simulink model "ssTest1"  (R2023b)
settings: Solver=VariableStepAuto  StartTime=0.0  StopTime=10.0  RelTol=1e-3
values from neighbouring files (symbols this model uses):
  Ad1 = A    [cDQN.m]    (also in ssTest.m = INVR*(I+A*dt/2))
  B = A*X    [Copy_of_cDQN.m]    (also in cCOM.m; cDQN.m)
  Bd1 = B    [cDQN.m]    (also in ssTest.m = INVR*B*dt/2)
  C = obj.fCalcMat(X(1)+1i*X(2) , B(1)+1i*B(2))    [Copy_of_cDQN.m]    (also in cCOM.m; cDQN.m)
  Cd1 = C    [cDQN.m]    (also in ssTest.m = C*Ad1)
  Dd11 = C*INVR*B*dt/2+D    [ssTest.m]
  Dd12 = C*INVR*B*dt/2    [ssTest.m]
undefined symbols (not defined in the file or in its folder): A, Ad2, Ad3, Bd2, Bd3, Cd21, Cd22, Cd3, D, Dd2, Dd3, Ts
libraries: DQN_Lib x1, spspowerguiLib x1
settings Model: Creator=rober  LastModifiedBy=rober

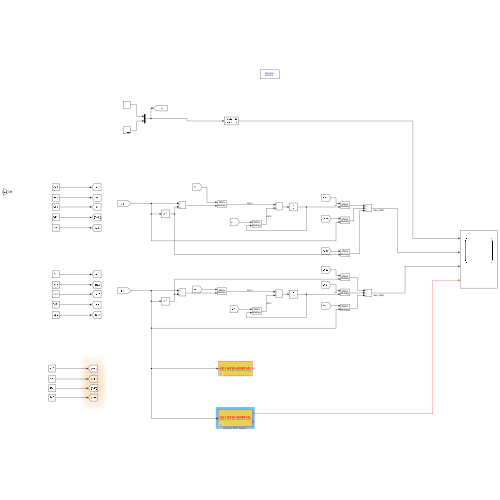
[thumbnail: Simulink's stored preview of the top-level diagram]
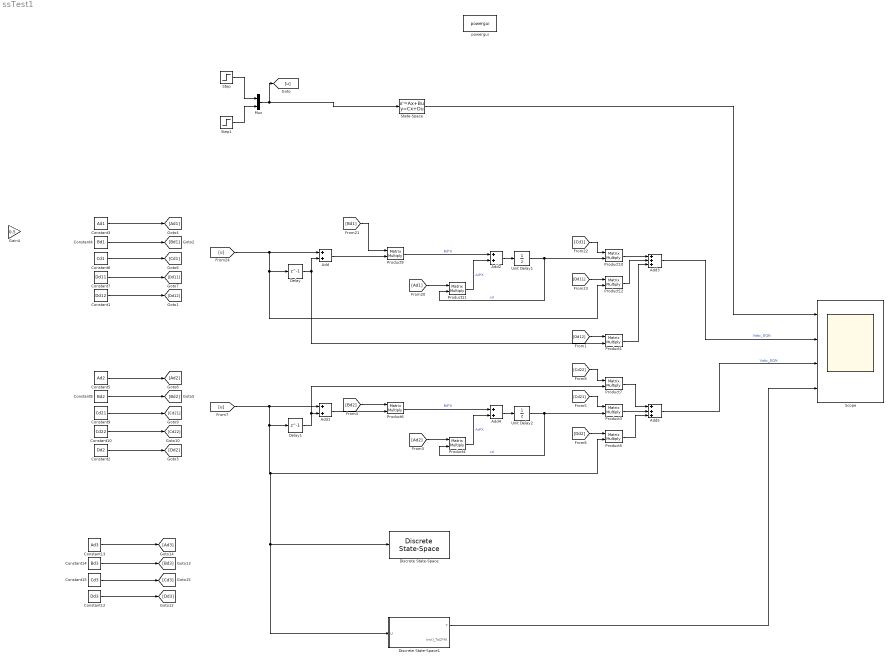
== system ssTest1 ==
  Add{,1..2,4} (4 alike) : Sum
  Add3 : Sum  Inputs=+++
  Add5 : Sum  Inputs=+++
  Constant1 : Constant  Value=Dd12
  Constant10 : Constant  Value=Cd22
  Constant12 : Constant  Value=Dd3
  Constant13 : Constant  Value=Ad3
  Constant14 : Constant  Value=Bd3
  Constant15 : Constant  Value=Cd3
  Constant2 : Constant  Value=Dd2
  Constant3 : Constant  Value=Ad1
  Constant4 : Constant  Value=Bd1
  Constant5 : Constant  Value=Ad2
  Constant6 : Constant  Value=Cd1
  Constant7 : Constant  Value=Dd11
  Constant8 : Constant  Value=Bd2
  Constant9 : Constant  Value=Cd21
  Delay : Delay  DelayLength=1  SampleTime=Ts
  Delay1 : Delay  DelayLength=1  SampleTime=Ts
  Discrete State-Space : DQN_Lib/Discrete State-Space  A=A  B=B  C=C  D=D  InitVec=0  dt=Ts
      settings: LibrarySourceBlock=|
      | spsSynchronousMachineModel/Discrete robust/State Space Model/Discretize
      | BE or Tustin
  Discrete State-Space1 : Subsystem  mask{A=A, B=B, C=C, D=D, InitVec=0, dt=Ts}
      mask prompts: InitVec "Initial condition:"; dt "Time step (s):"
      mask init:
      | I = eye(size(A,1));
      | INVR = I/(I-A*dt/2);
      | Ad1 = INVR*(I+A*dt/2);
      | Bd1 = INVR*B*dt/2;
      | Cd1 = C*Ad1;
      | Dd11 = C*INVR*B*dt/2+D;
      | Dd12 = C*INVR*B*dt/2;
      settings: LibrarySourceBlock=|
      | spsSynchronousMachineModel/Discrete robust/State Space Model/Discretize
      | BE or Tustin
      mask Display: disp(['{\color{red}\bf\fontsize{12}x(t) = Ad*x(t-dt)+Bd*u(t)}',newline,'{\color{gray}\bf\fontsize{12}y(t) = Cd*x(t-dt)+Dd*u(t)}'], 'texmode','on');
  Gain4 : Gain  Gain=0.5
  Mux : Mux  Inputs=2
  Product{1,3..7,9..12} (10 alike) : Product  Multiplication=Matrix(*)  SaturateOnIntegerOverflow=on  OutDataTypeStr=Inherit: Same as first input
  Scope : Scope  NumInputPorts=4
  State-Space : StateSpace  A=A  B=B  C=C  D=D  InitialCondition=0
  Step : Step  Time=3  Before=-0.668  After=5.668  SampleTime=Ts
  Step1 : Step  Time=8  Before=3.668  After=1.854  SampleTime=Ts
  Unit Delay1 : UnitDelay  SampleTime=Ts  HasFrameUpgradeWarning=on
  Unit Delay2 : UnitDelay  SampleTime=Ts  HasFrameUpgradeWarning=on
  powergui : spspowerguiLib/powergui  Priority=1  SimulationMode=Discrete  SampleTime=Ts  frequency=60  Iterations=50  frequencyindice=60  Pbase=100e6  ErrMax=1e-4  UnitsV=kV  UnitsW=MW  buscounter=0  FunctionMessages=off  echomessages=off  EnableUseOfTLC=off  CurrentSourceSwitches=off  DisableSnubberDevices=off  DisableRonSwitches=off  DisableVfSwitches=off  DisplayEquations=off  AutomaticDiscreteSolvers=off  SolverType=Tustin/Backward Euler (TBE)  Interpol=off  ExternalGateDelay=off  methode=off  Ts=100  x0status=blocks  SPID=on  SwTol=0  HookPort=off  NonlinearTolerance=1e-4  nMaxIteration=100  ContinueOnMaxIteration=off  RestoreLinks=warning  ResistiveCurrentMeasurement=off  Frange=[0:2:500]  Ylog=off  Xlog=on  ShowGrid=off  save=off  variable=ZData  structure=0  ZoomFFT=off  StartTime=0.0  cycles=1  DisplayStyle=1  fundamental=60  FreqAxis=off  MaxFrequency=1000  frequencyindicesteady=1  RmsSteady=1  display=off
  wires:
  Mux/1 -> [u], State-Space/1
  Step/1 -> Mux/1
  Step1/1 -> Mux/2
  State-Space/1 -> Scope/1
  Product10/1 -> Add3/1
  [Cd1] -> Product10/1
  Add/1 -> Product9/2
  Constant6/1 -> [Cd1]
  Unit Delay1/1 -> Product11/2, Product10/2  "xd"
  [Bd1] -> Product9/1
  Product11/1 -> Add2/2  "Ad*X"
  Constant3/1 -> [Ad1]
  Add2/1 -> Unit Delay1/1
  [Ad1] -> Product11/1
  Constant7/1 -> [Dd11]
  [Dd11] -> Product12/1
  Constant4/1 -> [Bd1]
  Product9/1 -> Add2/1  "Bd*U"
  Add3/1 -> Scope/2  "Vabc_DQN"
  [Dd12] -> Product1/1
  Delay/1 -> Product1/2, Add/2
  Product12/1 -> Add3/2
  Constant1/1 -> [Dd12]
  [u] -> Add/1, Product12/2, Delay/1
  Product1/1 -> Add3/3
  Add5/1 -> Scope/3  "Vabc_DQN"
  Constant2/1 -> [Dd2]
  Product5/1 -> Add5/3
  Constant10/1 -> [Cd22]
  [Ad2] -> Product4/1
  Constant8/1 -> [Bd2]
  [Dd2] -> Product5/1
  [u] -> Add1/1, Discrete State-Space1/1(U), Discrete State-Space/1, Product5/2, Delay1/1
  [Bd2] -> Product6/1
  Add4/1 -> Unit Delay2/1
  Product6/1 -> Add4/1  "Bd*U"
  Product4/1 -> Add4/2  "Ad*X"
  Add1/1 -> Product6/2
  Product3/1 -> Add5/2
  Unit Delay2/1 -> Product4/2, Product3/2  "xd"
  [Cd21] -> Product3/1
  Constant5/1 -> [Ad2]
  Delay1/1 -> Product7/2, Add1/2
  Constant9/1 -> [Cd21]
  [Cd22] -> Product7/1
  Product7/1 -> Add5/1
  Constant15/1 -> [Cd3]
  Constant13/1 -> [Ad3]
  Constant12/1 -> [Dd3]
  Constant14/1 -> [Bd3]
  Discrete State-Space1/1(Y) -> Scope/4

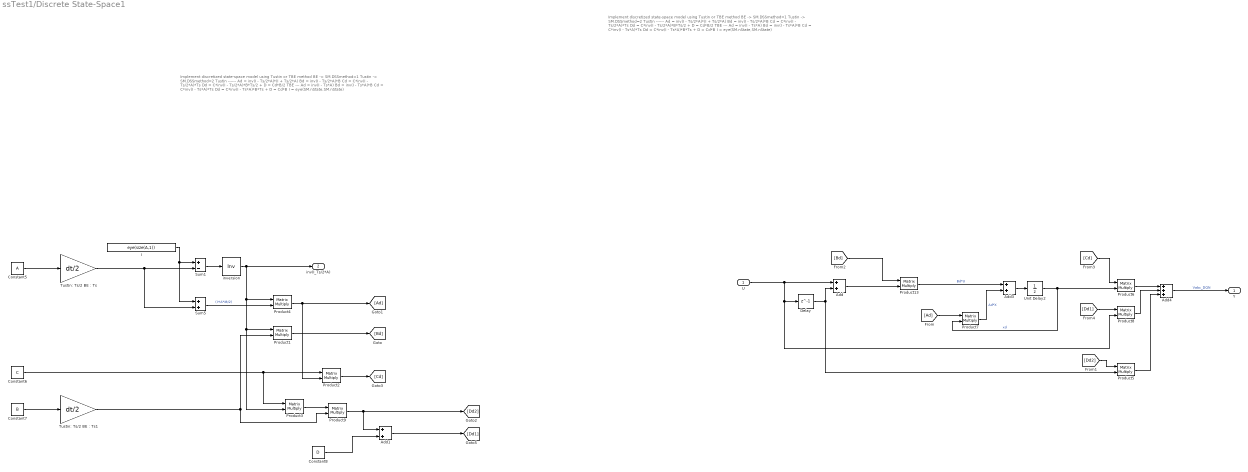
== system ssTest1/Discrete State-Space1 ==
  note: Implement discretized state-space model using Tustin or TBE method
      |
      | BE      -> SM.DSSmethod=1
      | Tustin  -> SM.DSSmethod=2
      |
      |
      | Tustin
      | ------
      | Ad = inv(I - Ts/2*A)*(I + Ts/2*A)
      | Bd = inv(I - Ts/2*A)*B
      | Cd = C*inv(I - Ts/2*A)*Ts
      | Dd = C*inv(I - Ts/2*A)*B*Ts/2  + D  =  Cd*B/2
      |
      | TBE
      | ---
      | Ad = inv(I - Ts*A)
      | Bd = inv(I - Ts*A)*B
      | Cd = C*inv(I - Ts*A)*Ts
      | Dd = C*inv(I - Ts*A)*B*Ts  + D  =  Cd*B
      |
      | I = eye(SM.nState,SM.nState)
  note: Implement discretized state-space model using Tustin or TBE method
      |
      | BE      -> SM.DSSmethod=1
      | Tustin  -> SM.DSSmethod=2
      |
      |
      | Tustin
      | ------
      | Ad = inv(I - Ts/2*A)*(I + Ts/2*A)
      | Bd = inv(I - Ts/2*A)*B
      | Cd = C*inv(I - Ts/2*A)*Ts
      | Dd = C*inv(I - Ts/2*A)*B*Ts/2  + D  =  Cd*B/2
      |
      | TBE
      | ---
      | Ad = inv(I - Ts*A)
      | Bd = inv(I - Ts*A)*B
      | Cd = C*inv(I - Ts*A)*Ts
      | Dd = C*inv(I - Ts*A)*B*Ts  + D  =  Cd*B
      |
      | I = eye(SM.nState,SM.nState)
  U : Inport
  Add : Sum
  Add1 : Sum
  Add3 : Sum
  Add4 : Sum  Inputs=+++
  Constant5 : Constant  Value=A
  Constant6 : Constant  Value=C
  Constant7 : Constant  Value=B
  Constant8 : Constant  Value=D
  Delay : Delay  DelayLength=1  SampleTime=Ts
  I : Constant  Value=eye(size(A,1))
  Product{1..9,13} (10 alike) : Product  Multiplication=Matrix(*)  SaturateOnIntegerOverflow=on  OutDataTypeStr=Inherit: Same as first input
  Sum1 : Sum  Inputs=+-  SaturateOnIntegerOverflow=on
  Sum5 : Sum  SaturateOnIntegerOverflow=on
  "Tustin: Ts/2 BE : Ts" : Gain  Gain=dt/2  SaturateOnIntegerOverflow=on  OutDataTypeStr=Inherit: Same as input  ParamDataTypeStr=Inherit: Same as input
  "Tustin: Ts/2 BE : Ts1" : Gain  Gain=dt/2  SaturateOnIntegerOverflow=on  OutDataTypeStr=Inherit: Same as input  ParamDataTypeStr=Inherit: Same as input
  Unit Delay2 : UnitDelay  InitialCondition=InitVec  SampleTime=dt  HasFrameUpgradeWarning=on
  inversion : Product  Inputs=/  Multiplication=Matrix(*)  RndMeth=Zero
  Y : Outport
  inv(I_Ts/2*A) : Outport  Port=2  VectorParamsAs1DForOutWhenUnconnected=off
  wires:
  Add4/1 -> Y/1  "Vabc_DQN"
  [Dd2] -> Product5/1
  Product5/1 -> Add4/3
  Product8/1 -> Add4/2
  [Ad] -> Product7/1
  [Dd1] -> Product8/1
  U/1 -> Add/1, Product8/2, Delay/1
  [Bd] -> Product13/1
  Product13/1 -> Add3/1  "Bd*U"
  Product7/1 -> Add3/2  "Ad*X"
  Add/1 -> Product13/2
  Product6/1 -> Add4/1
  Unit Delay2/1 -> Product7/2, Product6/2  "xd"
  [Cd] -> Product6/1
  Delay/1 -> Product5/2, Add/2
  Add3/1 -> Unit Delay2/1
  Product4/1 -> Product2/2, [Ad]
  Add1/1 -> [Dd1]
  Product1/1 -> [Bd]
  Sum5/1 -> Product4/2  "(I+A*dt/2)"
  Constant7/1 -> "Tustin: Ts/2 BE : Ts1"/1
  Constant6/1 -> Product3/1, Product2/1
  Product2/1 -> [Cd]
  inversion/1 -> Product3/2, Product1/1, Product4/1, inv(I_Ts/2*A)/1
  Sum1/1 -> inversion/1
  "Tustin: Ts/2 BE : Ts"/1 -> Sum1/2, Sum5/2
  Constant5/1 -> "Tustin: Ts/2 BE : Ts"/1
  I/1 -> Sum5/1, Sum1/1
  "Tustin: Ts/2 BE : Ts1"/1 -> Product9/2, Product1/2
  Product3/1 -> Product9/1
  Product9/1 -> [Dd2], Add1/1
  Constant8/1 -> Add1/2
